simulink model "recti_feedback_ctrl2"  (Simulink 9.1)
settings: Solver=ode4  StartTime=0.0  StopTime=5  FixedStep=0.001  RelTol=1e-3
settings Model: Creator=HuuNgan  LastModifiedBy=HuuNgan
settings DataIOCC: SaveFormat=Dataset
settings OptimizationCC: LifeSpan=auto
settings DebuggingCC: UnderspecifiedInitializationDetection=Simplified  MergeDetectMultiDrivingBlocksExec=error  SFUnexpectedBacktrackingDiag=error  SFNoUnconditionalDefaultTransitionDiag=error  SFExecutionAtInitializationDiag=warning
settings HardwareCC: ProdBitPerPointer=64  ProdBitPerSizeT=64  ProdBitPerPtrDiffT=64  ProdLargestAtomicFloat=Float  ProdIntDivRoundTo=Zero  ProdEndianess=LittleEndian  ProdWordSize=64  ProdHWDeviceType=Intel->x86-64 (Windows64)
settings ModelReferenceCC: PropagateSignalLabelsOutOfModel=on
settings CodeAppCC: StateflowObjectComments=off
settings GRTTargetCC: TargetLangStandard=C99 (ISO)  CombineOutputUpdateFcns=on  GRTInterface=off
settings ConfigComp: CovMetricSettings=dwe  CovHtmlReporting=off  CovSaveCumulativeToWorkspaceVar=off  CovSaveSingleToWorkspaceVar=off  CovExternalEMLEnable=on

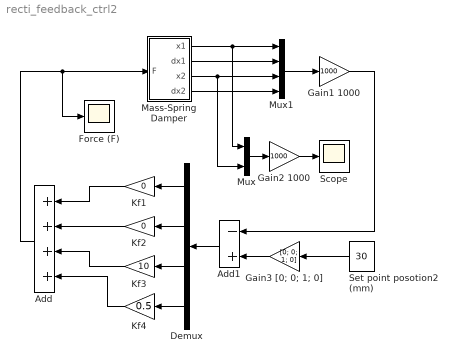
== system recti_feedback_ctrl2 ==
  "Add " : Sum  Inputs=++++
  "Add1 " : Sum  Inputs=-+
  Demux : Demux
  Force (F) : Scope
  Gain1 1000 : Gain  Gain=1000
  "Gain2 1000 " : Gain  Gain=1000
  Gain3 [0; 0; 1; 0] : Gain  Gain=[0; 0; 1; 0]
  Kf1 : Gain  Gain=0
  Kf2 : Gain  Gain=0
  Kf3 : Gain  Gain=10
  Kf4 : Gain  Gain=0.5
  Mass-Spring Damper : Subsystem
  Mux : Mux  Inputs=2
  Mux1 : Mux
  "Scope " : Scope
  Set point posotion2 (mm) : Constant  Value=30  SampleTime=0.001
  wires:
  Mass-Spring Damper/1(x1) -> Mux1/1, Mux/1
  Mass-Spring Damper/2(dx1) -> Mux1/2
  Mass-Spring Damper/4(dx2) -> Mux1/4
  Mass-Spring Damper/3(x2) -> Mux1/3, Mux/2
  Mux1/1 -> Gain1 1000/1
  Mux/1 -> "Gain2 1000 "/1
  "Gain2 1000 "/1 -> "Scope "/1
  Set point posotion2 (mm)/1 -> Gain3 [0; 0; 1; 0]/1
  Gain3 [0; 0; 1; 0]/1 -> "Add1 "/2
  Gain1 1000/1 -> "Add1 "/1
  "Add1 "/1 -> Demux/1
  Demux/1 -> Kf1/1
  Demux/2 -> Kf2/1
  Demux/3 -> Kf3/1
  Demux/4 -> Kf4/1
  Kf1/1 -> "Add "/1
  Kf2/1 -> "Add "/2
  Kf3/1 -> "Add "/3
  Kf4/1 -> "Add "/4
  "Add "/1 -> Force (F)/1, Mass-Spring Damper/1(F)

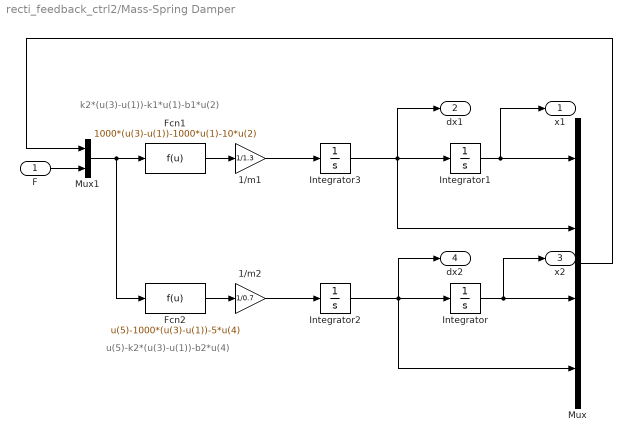
== system recti_feedback_ctrl2/Mass-Spring Damper ==
  note: u(5)-k2*(u(3)-u(1))-b2*u(4)
  note: k2*(u(3)-u(1))-k1*u(1)-b1*u(2)
  F : Inport
  1/m1 : Gain  Gain=1/1.3
  1/m2 : Gain  Gain=1/0.7
  "Fcn1 " : Fcn  Expr=1000*(u(3)-u(1))-1000*u(1)-10*u(2)
  "Fcn2 " : Fcn  Expr=u(5)-1000*(u(3)-u(1))-5*u(4)
  Integrator{,1..3} (4 alike) : Integrator
  Mux : Mux
  Mux1 : Mux  Inputs=2
  x1 : Outport
  dx1 : Outport  Port=2
  x2 : Outport  Port=3
  dx2 : Outport  Port=4
  wires:
  Integrator3/1 -> dx1/1, Mux/2, Integrator1/1
  Mux1/1 -> "Fcn2 "/1, "Fcn1 "/1
  "Fcn2 "/1 -> 1/m2/1
  Integrator/1 -> x2/1, Mux/3
  1/m2/1 -> Integrator2/1
  F/1 -> Mux1/2
  1/m1/1 -> Integrator3/1
  Integrator1/1 -> x1/1, Mux/1
  Integrator2/1 -> dx2/1, Mux/4, Integrator/1
  Mux/1 -> Mux1/1
  "Fcn1 "/1 -> 1/m1/1
